simulink model "buildingEnergyManagement"  (R2019b)
settings: Solver=FixedStepAuto  StartTime=0.0  StopTime=24  FixedStep=1/12  RelTol=1e-3  AbsTol=1e-6
values from neighbouring files (symbols this model uses):
  c = 1005.4    [init_vars.m]
  cost = 0.09/3.6e6    (= 2.5e-08)    [init_vars.m]
  eta_ac = 0.85    [init_vars.m]
  initToutdoor = 60    [bonsaiAssess.m]    (also in bonsaiExportConnect.m; bonsaiPredict.m; run_benchmark.m = 30)
  Mdot = 3600    [init_vars.m]
  THeater = 50    [init_vars.m]
  TinIC = 20    [init_vars.m]
undefined symbols (not defined in the file or in its folder): dTac, n_rooms, nWindows_room1, nWindows_room2, nWindows_room3, sigbuilder_block
libraries: simulink_extras x7, bonsai_library x1
Description:
  | Thermal Model of a House
  | 
  | This demo illustrates how you can use Simulink(R) to create the thermal model of
  | a house. This system models the outdoor environment, the thermal
  | characteristics of the house, and the house heating system.
  | 
  | The sldemo_househeat_data.m file initializes data in the model workspace.
  | To make changes, you can edit the model workspace directly or edit the MATLAB(R) file
  | and re-load the model workspace.
  | 
  | To view the model workspace, select View > Model Explorer
  | from the Simulink editor.
  | 
  | Note: Time is given in units of hours
settings Model: ExtModeTrigMode=oneshot  ExtModeArmWhenConnect=off  ExtModeAutoUpdateStatusClock=off  OrderedModelArguments=off  Creator=The MathWorks, Inc.  LastModifiedBy=jomcdowe
settings SolverCC: AutoScaleAbsTol=off
settings DataIOCC: ExternalInput=[]  InitialState=[]  SaveOutput=off  ReturnWorkspaceOutputs=off  SignalLoggingName=sldemo_househeat_output  ReturnWorkspaceOutputsName=simout
settings OptimizationCC: BlockReduction=off  BooleanDataType=off  ExpressionDepthLimit=2147483647  InitFltsAndDblsToZero=on  LifeSpan=inf  BufferReusableBoundary=off
settings DebuggingCC: SaveWithParameterizedLinksMsg=none  UnderspecifiedInitializationDetection=Classic  MergeDetectMultiDrivingBlocksExec=none  SignalResolutionControl=TryResolveAllWithWarning  MultiTaskDSMMsg=warning  MultiTaskCondExecSysMsg=none  IntegerOverflowMsg=none  FcnCallInpInsideContextMsg=warning  BusObjectLabelMismatch=none  StateNameClashWarn=warning  SFUnexpectedBacktrackingDiag=warning  SFNoUnconditionalDefaultTransitionDiag=warning  SFExecutionAtInitializationDiag=none  IntegerSaturationMsg=none  ArithmeticOperatorsInVariantConditions=warning
settings HardwareCC: ProdBitPerPointer=32  ProdBitPerSizeT=32  ProdBitPerPtrDiffT=32  ProdLargestAtomicFloat=None  ProdIntDivRoundTo=Undefined  ProdEndianess=Unspecified  ProdWordSize=32  ProdHWDeviceType=32-bit Generic  TargetUnknown=on
settings ModelReferenceCC: PropagateSignalLabelsOutOfModel=off
settings SFSimCC: SimUseLocalCustomCode=off  CustomCodeUndefinedFunction=UseInterfaceOnly
settings RTWCC: Description=Generic Real-Time Target  RTWUseLocalCustomCode=off
settings CodeAppCC: StateflowObjectComments=on
settings GRTTargetCC: TargetFcnLib=ansi_tfl_tmw.mat  TargetLangStandard=C89/C90 (ANSI)  CombineOutputUpdateFcns=off  GRTInterface=on
settings ConfigComp: CovMetricSettings=dw  CovSaveCumulativeToWorkspaceVar=on  CovSaveSingleToWorkspaceVar=on  CovExternalEMLEnable=off

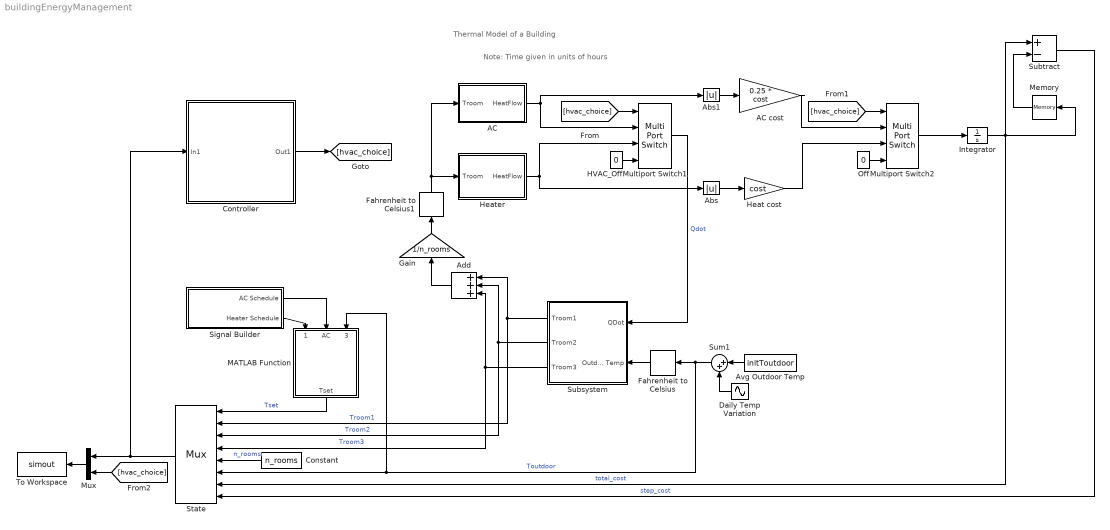
== system buildingEnergyManagement ==
  note: Thermal Model of a Building
  note: Note: Time given in units of hours
  AC : Subsystem
  AC cost : Gain  Gain=0.25 * cost  SaturateOnIntegerOverflow=on  OutDataTypeStr=Inherit: Same as input  ParamDataTypeStr=Inherit: Same as input
  Abs : Abs
  Abs1 : Abs
  Add : Sum  Inputs=+++
  Avg Outdoor Temp : Constant  Value=initToutdoor
  Constant : Constant  Value=n_rooms
  Controller : Subsystem  VariantControlMode=Label  Variant=on  LabelModeActiveChoice=Bonsai  mask{VChoice=Bonsai}
      mask prompts: VChoice "Source"
      mask init:
      | simulationStatus =  get_param(bdroot,'SimulationStatus');
      | 
      | % The active variant can only be modified at edit-time or very early during
      | % the simulink compile stage. 
      | 
      |     choice = get_param(gcb,'VChoice');
      |     vssBlk = gcb;
      |     oldVariant = get_param(gcb,'OverrideUsingVariant');
      | 
      |     if strcmp(choice,'Thermostat')
      |         set_param(vssBlk, 'OverrideUsingVariant', 'Thermostat');
      |     else
      |         set_param(vssBlk, 'OverrideUsingVariant', 'Bonsai');
      |     end
      mask TypeOptions VChoice: Thermostat | Bonsai
      mask Display:
      | choice = get_param(gcb,'VChoice');
      | 
      | if strcmp(choice,'Thermostat')
      |     image('img/Thermostat.jpg');
      | else
      |     image('img/Bonsai.jpg');
      | end
  Daily Temp Variation : Sin  Amplitude=15  Frequency=2*pi/24  SampleTime=0
  Fahrenheit to Celsius : simulink_extras/Transformations/Fahrenheit to Celsius
      settings: SourceProductName=Simulink Extras
  Fahrenheit to Celsius1 : simulink_extras/Transformations/Fahrenheit to Celsius
      settings: SourceProductBaseCode=SL
  Gain : Gain  Gain=1/n_rooms
  HVAC_Off : Constant  Value=0
  "Heat cost " : Gain  Gain=cost  SaturateOnIntegerOverflow=on  OutDataTypeStr=Inherit: Same as input  ParamDataTypeStr=Inherit: Same as input
  Heater : Subsystem
  Integrator : Integrator
  MATLAB Function : MATLAB Function  TreatAsAtomicUnit=on
  Memory : Memory
  Multiport Switch1 : MultiPortSwitch  DiagnosticForDefault=None
  Multiport Switch2 : MultiPortSwitch  DiagnosticForDefault=None
  Mux : Mux  Inputs=2
  Off : Constant  Value=0
  Signal Builder : Subsystem  Tag=STV Subsys  LoadFcn=sigbuilder_block('load');  StartFcn=sigbuilder_block('start');  StopFcn=sigbuilder_block('stop');  ClipboardFcn=sigbuilder_block('clipboard');  mask(Sigbuilder block){tuvar=[0:10]}
      mask help: Simulink:masks:SigbuilderBlock_MD
      mask init:
      | if ~strcmp(get_param(bdroot(gcbh),'SimulationStatus'),'stopped') tuvar = sigbuilder_block('maskInit'); end
      settings: CopyFcn=sigbuilder_block('copy');  DeleteFcn=sigbuilder_block('delete');  ModelCloseFcn=sigbuilder_block('modelClose');  PreSaveFcn=sigbuilder_block('preSave');  PauseFcn=sigbuilder_block('pause');  ContinueFcn=sigbuilder_block('continue');  NameChangeFcn=sigbuilder_block('namechange');  OpenFcn=sigbuilder_block('open',[437.6 199.2 550.4 400 ]);  CloseFcn=sigbuilder_block('close');
      mask Display: plot(0, 0, 100, 100,[2, 2, 32, 32, 2], [68, 8, 8, 68, 68],[32, 2], [38, 38], [32, 19, 2],[53, 60, 44], [32, 17, 17, 2],[16, 16, 31, 31]);txt = getActiveGroup(gcbh);text(2, 100, txt,'verticalAlignment', 'top');
  State : Mux  Inputs=8
      settings: DisplayOption=signals
  Subsystem : Subsystem
  Subtract : Sum  Inputs=+-
  Sum1 : Sum  Inputs=|++  SaturateOnIntegerOverflow=on  InputSameDT=on  OutDataTypeStr=Inherit: Same as first input
  To Workspace : ToWorkspace  VariableName=simout  SampleTime=-1
  wires:
  Sum1/1 -> State/6, MATLAB Function/3(Toutdoor), Fahrenheit to Celsius/1  "Toutdoor"
  Avg Outdoor Temp/1 -> Sum1/1
  Daily Temp Variation/1 -> Sum1/2
  HVAC_Off/1 -> Multiport Switch1/4
  [hvac_choice] -> Multiport Switch1/1
  [hvac_choice] -> Multiport Switch2/1
  Off/1 -> Multiport Switch2/4
  AC/1(HeatFlow) -> Abs1/1, Multiport Switch1/2
  Heater/1(HeatFlow) -> Abs/1, Multiport Switch1/3
  Abs1/1 -> AC cost/1
  Abs/1 -> "Heat cost "/1
  AC cost/1 -> Multiport Switch2/2
  "Heat cost "/1 -> Multiport Switch2/3
  Controller/1(Out1) -> [hvac_choice]
  [hvac_choice] -> Mux/2
  Mux/1 -> To Workspace/1
  Signal Builder/2(Heater Schedule) -> MATLAB Function/1(Heater)
  Signal Builder/1(AC Schedule) -> MATLAB Function/2(AC)
  Multiport Switch1/1 -> Subsystem/1(QDot)  "Qdot"
  Fahrenheit to Celsius/1 -> Subsystem/2(Outdoor Temp)
  State/1 -> Mux/1, Controller/1(In1)
  MATLAB Function/1(Tset) -> State/1  "Tset"
  Integrator/1 -> Memory/1, State/7, Subtract/1  "total_cost"
  Subsystem/1(Troom1) -> Add/1, State/2  "Troom1"
  Subsystem/2(Troom2) -> Add/2, State/3  "Troom2"
  Subsystem/3(Troom3) -> Add/3, State/4  "Troom3"
  Add/1 -> Gain/1
  Fahrenheit to Celsius1/1 -> AC/1(Troom), Heater/1(Troom)
  Gain/1 -> Fahrenheit to Celsius1/1
  Constant/1 -> State/5  "n_rooms"
  Multiport Switch2/1 -> Integrator/1
  Memory/1 -> Subtract/2
  Subtract/1 -> State/8  "step_cost"

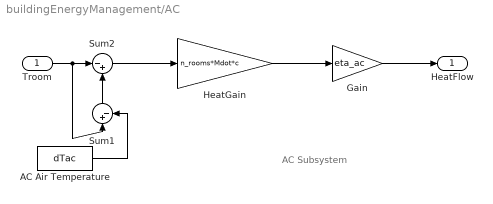
== system buildingEnergyManagement/AC ==
  note: AC Subsystem
  Troom : Inport
  AC Air Temperature : Constant  Value=dTac
  Gain : Gain  Gain=eta_ac
  HeatGain : Gain  Gain=n_rooms*Mdot*c
  Sum1 : Sum  Inputs=|+-
  Sum2 : Sum  Inputs=|-+
  HeatFlow : Outport  VectorParamsAs1DForOutWhenUnconnected=off
  wires:
  Sum2/1 -> HeatGain/1
  Gain/1 -> HeatFlow/1
  HeatGain/1 -> Gain/1
  AC Air Temperature/1 -> Sum1/2
  Troom/1 -> Sum2/1, Sum1/1
  Sum1/1 -> Sum2/2

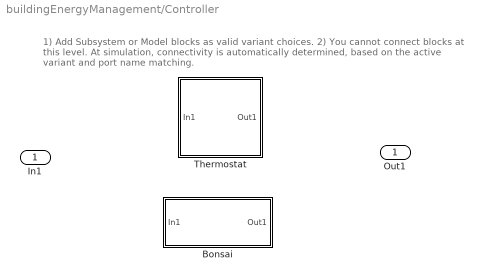
== system buildingEnergyManagement/Controller ==
  note: 1) Add Subsystem or Model blocks as valid variant choices.
      | 2) You cannot connect blocks at this level. At simulation, connectivity is automatically
      | determined, based on the active variant and port name matching.
  In1 : Inport
  Bonsai : Subsystem  VariantControl=Bonsai
  Thermostat : Subsystem  VariantControl=Thermostat
      mask Display: image(fullfile(matlabroot,'toolbox','simulink','simdemos','simgeneral','images','HouseHeatThermostatPix.svg'))
  Out1 : Outport

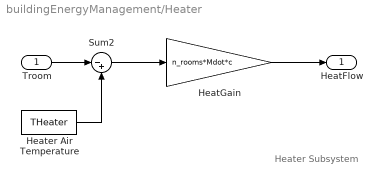
== system buildingEnergyManagement/Heater ==
  note: Heater Subsystem
  Troom : Inport
  HeatGain : Gain  Gain=n_rooms*Mdot*c
  Heater Air Temperature : Constant  Value=THeater
  Sum2 : Sum  Inputs=|-+
  HeatFlow : Outport  VectorParamsAs1DForOutWhenUnconnected=off
  wires:
  Heater Air Temperature/1 -> Sum2/2
  Troom/1 -> Sum2/1
  Sum2/1 -> HeatGain/1
  HeatGain/1 -> HeatFlow/1

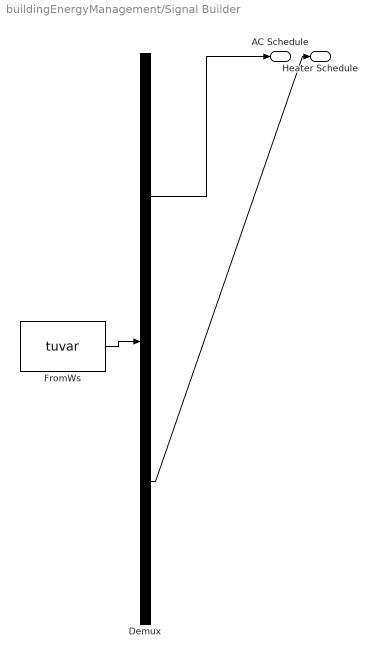
== system buildingEnergyManagement/Signal Builder ==
  Demux : Demux  Tag=STV Demux  Outputs=2
  FromWs : FromWorkspace  Tag=STV FromWs  VariableName=tuvar  SampleTime=0
      SigBuilderData=|
      | common.afterFinalStr = 'Extrapolate'
      | common.sampleTime = 0
      | dataSet.timeRange = [0 24]
      | dataSet.name = 'Tset_choice'
      | sbobj.Groups.Name = 'Tset_choice'
      | sbobj.Groups.Signals(1).Name = 'AC Schedule'
      | sbobj.Groups.Signals(1).XData = [0 12 12 24]
      | sbobj.Groups.Signals(1).YData = [78 78 86 86]
      | sbobj.Groups.Signals(2).Name = 'Heater Schedule'
      | sbobj.Groups.Signals(2).XData = [0 12 12 24]
      | sbobj.Groups.Signals(2).YData = [68 68 60 60]
      | sbobj.Groups.TimeRange = [0 24]
  AC Schedule : Outport  Tag=STV Outport
  Heater Schedule : Outport  Tag=STV Outport  Port=2
  wires:
  Demux/1 -> AC Schedule/1
  FromWs/1 -> Demux/1
  Demux/2 -> Heater Schedule/1

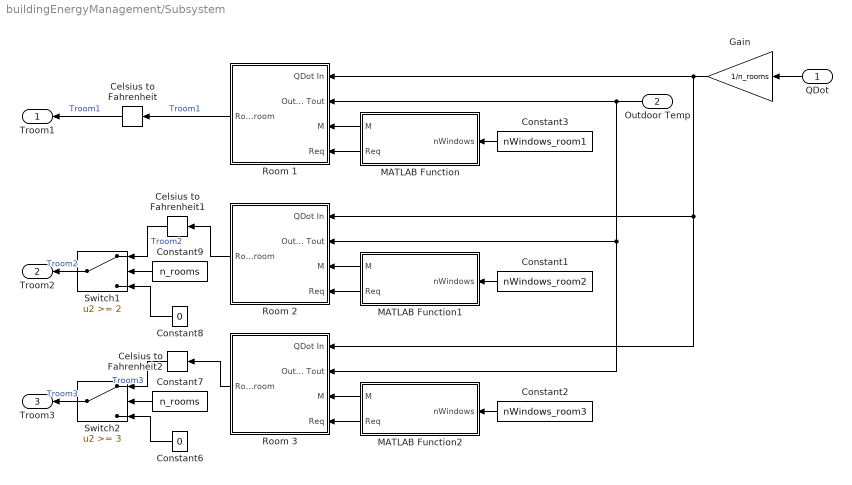
== system buildingEnergyManagement/Subsystem ==
  QDot : Inport
  Outdoor Temp : Inport  Port=2
  Celsius to Fahrenheit : simulink_extras/Transformations/Celsius to Fahrenheit
      settings: SourceProductName=Simulink Extras
  Celsius to Fahrenheit1 : simulink_extras/Transformations/Celsius to Fahrenheit
      settings: SourceProductName=Simulink Extras
  Celsius to Fahrenheit2 : simulink_extras/Transformations/Celsius to Fahrenheit
      settings: SourceProductName=Simulink Extras
  Constant1 : Constant  Value=nWindows_room2  VectorParams1D=off
  Constant2 : Constant  Value=nWindows_room3  VectorParams1D=off
  Constant3 : Constant  Value=nWindows_room1  VectorParams1D=off
  Constant6 : Constant  Value=0
  Constant7 : Constant  Value=n_rooms
  Constant8 : Constant  Value=0
  Constant9 : Constant  Value=n_rooms
  Gain : Gain  Gain=1/n_rooms
  MATLAB Function : MATLAB Function  TreatAsAtomicUnit=on
  MATLAB Function1 : MATLAB Function  TreatAsAtomicUnit=on
  MATLAB Function2 : MATLAB Function  TreatAsAtomicUnit=on
  Room 1 : Subsystem
      mask Display: image(fullfile(matlabroot,'toolbox','simulink','simdemos','simgeneral','images','HouseHeatHousePix.svg'))
  Room 2 : Subsystem
      mask Display: image(fullfile(matlabroot,'toolbox','simulink','simdemos','simgeneral','images','HouseHeatHousePix.svg'))
  Room 3 : Subsystem
      mask Display: image(fullfile(matlabroot,'toolbox','simulink','simdemos','simgeneral','images','HouseHeatHousePix.svg'))
  Switch1 : Switch  Threshold=2
  Switch2 : Switch  Threshold=3
  Troom1 : Outport
  Troom2 : Outport  Port=2
  Troom3 : Outport  Port=3
  wires:
  Gain/1 -> Room 1/1(QDot In), Room 2/1(QDot In), Room 3/1(QDot In)
  Outdoor Temp/1 -> Room 1/2(Outdoor Temp Tout), Room 2/2(Outdoor Temp Tout), Room 3/2(Outdoor Temp Tout)
  QDot/1 -> Gain/1
  Constant9/1 -> Switch1/2
  Room 2/1(Room Temp Troom) -> Celsius to Fahrenheit1/1
  Constant7/1 -> Switch2/2
  Room 3/1(Room Temp Troom) -> Celsius to Fahrenheit2/1
  Switch2/1 -> Troom3/1  "Troom3"
  Switch1/1 -> Troom2/1  "Troom2"
  Room 1/1(Room Temp Troom) -> Celsius to Fahrenheit/1  "Troom1"
  Celsius to Fahrenheit/1 -> Troom1/1  "Troom1"
  Constant8/1 -> Switch1/3
  Celsius to Fahrenheit1/1 -> Switch1/1  "Troom2"
  Celsius to Fahrenheit2/1 -> Switch2/1  "Troom3"
  Constant6/1 -> Switch2/3
  MATLAB Function/1(M) -> Room 1/3(M)
  MATLAB Function/2(Req) -> Room 1/4(Req)
  Constant3/1 -> MATLAB Function/1(nWindows)
  MATLAB Function1/1(M) -> Room 2/3(M)
  MATLAB Function1/2(Req) -> Room 2/4(Req)
  Constant1/1 -> MATLAB Function1/1(nWindows)
  MATLAB Function2/1(M) -> Room 3/3(M)
  MATLAB Function2/2(Req) -> Room 3/4(Req)
  Constant2/1 -> MATLAB Function2/1(nWindows)

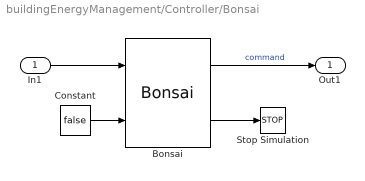
== system buildingEnergyManagement/Controller/Bonsai ==
  In1 : Inport
  Bonsai : bonsai_library/Bonsai  sampleTime=[-1, 0]
      settings: SourceProductName=Bonsai Toolbox
  Constant : Constant  Value=false
  Stop Simulation : Stop
  Out1 : Outport
  wires:
  Bonsai/1 -> Out1/1  "command"
  In1/1 -> Bonsai/1
  Constant/1 -> Bonsai/2
  Bonsai/2 -> Stop Simulation/1

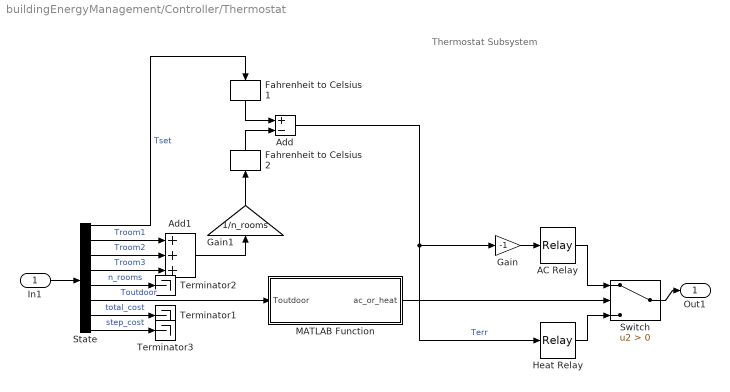
== system buildingEnergyManagement/Controller/Thermostat ==
  note: Thermostat Subsystem
  In1 : Inport
  AC Relay : Relay  OnSwitchValue=5*(5/9)  OffSwitchValue=-5*(5/9)  OffOutputValue=3
  Add : Sum  Inputs=+-
  Add1 : Sum  Inputs=+++
  Fahrenheit to Celsius 1 : simulink_extras/Transformations/Fahrenheit to Celsius
      settings: SourceProductName=Simulink Extras
  Fahrenheit to Celsius 2 : simulink_extras/Transformations/Fahrenheit to Celsius
      settings: SourceProductName=Simulink Extras
  Gain : Gain  Gain=-1
  Gain1 : Gain  Gain=1/n_rooms
  Heat Relay : Relay  OnSwitchValue=5*(5/9)  OffSwitchValue=-5*(5/9)  OnOutputValue=2  OffOutputValue=3
  MATLAB Function : MATLAB Function  TreatAsAtomicUnit=on
  State : Demux  Outputs=8
  Switch : Switch  Criteria=u2 > Threshold
  Terminator1 : Terminator
  Terminator2 : Terminator
  Terminator3 : Terminator
  Out1 : Outport
  wires:
  Add/1 -> Heat Relay/1, Gain/1  "Terr"
  MATLAB Function/1(ac_or_heat) -> Switch/2
  Heat Relay/1 -> Switch/3
  AC Relay/1 -> Switch/1
  Switch/1 -> Out1/1
  Gain/1 -> AC Relay/1
  Fahrenheit to Celsius 1/1 -> Add/1
  Fahrenheit to Celsius 2/1 -> Add/2
  In1/1 -> State/1
  State/1 -> Fahrenheit to Celsius 1/1  "Tset"
  State/3 -> Add1/2  "Troom2"
  State/4 -> Add1/3  "Troom3"
  State/2 -> Add1/1  "Troom1"
  Add1/1 -> Gain1/1
  Gain1/1 -> Fahrenheit to Celsius 2/1
  State/7 -> Terminator1/1  "total_cost"
  State/6 -> MATLAB Function/1(Toutdoor)  "Toutdoor"
  State/5 -> Terminator2/1  "n_rooms"
  State/8 -> Terminator3/1  "step_cost"

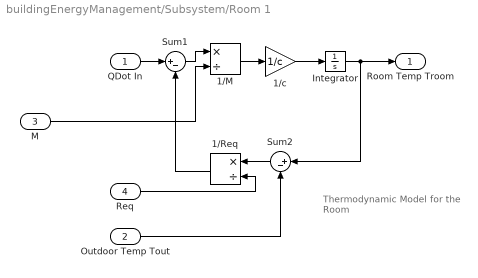
== system buildingEnergyManagement/Subsystem/Room 1 ==
  note: Thermodynamic Model
      | for the Room
  QDot In : Inport
  Outdoor Temp Tout : Inport  Port=2
  M : Inport  Port=3
  Req : Inport  Port=4
  1/M : Product  Inputs=*/
  1/Req : Product  Inputs=*/
  1/c : Gain  Gain=1/c  SaturateOnIntegerOverflow=on  OutDataTypeStr=Inherit: Same as input  ParamDataTypeStr=Inherit: Same as input
  Integrator : Integrator  InitialCondition=TinIC
  Sum1 : Sum  Inputs=|+-  SaturateOnIntegerOverflow=on  InputSameDT=on  OutDataTypeStr=Inherit: Same as first input
  Sum2 : Sum  Inputs=|+-  SaturateOnIntegerOverflow=on  InputSameDT=on  OutDataTypeStr=Inherit: Same as first input
  Room Temp Troom : Outport  InitialOutput=0  VectorParamsAs1DForOutWhenUnconnected=off
  wires:
  M/1 -> 1/M/2
  1/M/1 -> 1/c/1
  Sum1/1 -> 1/M/1
  Req/1 -> 1/Req/2
  Integrator/1 -> Room Temp Troom/1, Sum2/1
  1/c/1 -> Integrator/1
  1/Req/1 -> Sum1/2
  Sum2/1 -> 1/Req/1
  QDot In/1 -> Sum1/1
  Outdoor Temp Tout/1 -> Sum2/2

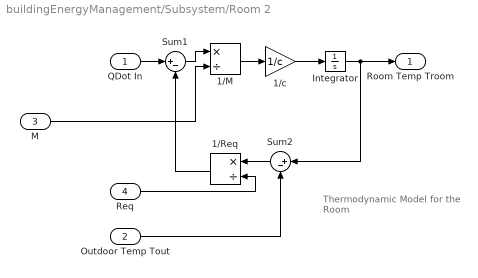
== system buildingEnergyManagement/Subsystem/Room 2 ==
  note: Thermodynamic Model
      | for the Room
  QDot In : Inport
  Outdoor Temp Tout : Inport  Port=2
  M : Inport  Port=3
  Req : Inport  Port=4
  1/M : Product  Inputs=*/
  1/Req : Product  Inputs=*/
  1/c : Gain  Gain=1/c  SaturateOnIntegerOverflow=on  OutDataTypeStr=Inherit: Same as input  ParamDataTypeStr=Inherit: Same as input
  Integrator : Integrator  InitialCondition=TinIC
  Sum1 : Sum  Inputs=|+-  SaturateOnIntegerOverflow=on  InputSameDT=on  OutDataTypeStr=Inherit: Same as first input
  Sum2 : Sum  Inputs=|+-  SaturateOnIntegerOverflow=on  InputSameDT=on  OutDataTypeStr=Inherit: Same as first input
  Room Temp Troom : Outport  InitialOutput=0  VectorParamsAs1DForOutWhenUnconnected=off
  wires:
  M/1 -> 1/M/2
  1/M/1 -> 1/c/1
  Sum1/1 -> 1/M/1
  Req/1 -> 1/Req/2
  Integrator/1 -> Room Temp Troom/1, Sum2/1
  1/c/1 -> Integrator/1
  1/Req/1 -> Sum1/2
  Sum2/1 -> 1/Req/1
  QDot In/1 -> Sum1/1
  Outdoor Temp Tout/1 -> Sum2/2

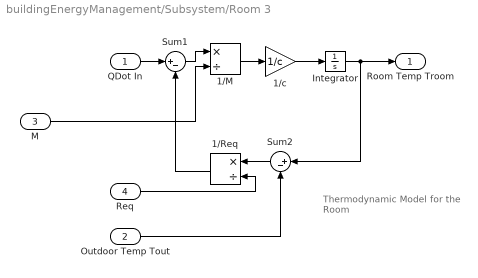
== system buildingEnergyManagement/Subsystem/Room 3 ==
  note: Thermodynamic Model
      | for the Room
  QDot In : Inport
  Outdoor Temp Tout : Inport  Port=2
  M : Inport  Port=3
  Req : Inport  Port=4
  1/M : Product  Inputs=*/
  1/Req : Product  Inputs=*/
  1/c : Gain  Gain=1/c  SaturateOnIntegerOverflow=on  OutDataTypeStr=Inherit: Same as input  ParamDataTypeStr=Inherit: Same as input
  Integrator : Integrator  InitialCondition=TinIC
  Sum1 : Sum  Inputs=|+-  SaturateOnIntegerOverflow=on  InputSameDT=on  OutDataTypeStr=Inherit: Same as first input
  Sum2 : Sum  Inputs=|+-  SaturateOnIntegerOverflow=on  InputSameDT=on  OutDataTypeStr=Inherit: Same as first input
  Room Temp Troom : Outport  InitialOutput=0  VectorParamsAs1DForOutWhenUnconnected=off
  wires:
  M/1 -> 1/M/2
  1/M/1 -> 1/c/1
  Sum1/1 -> 1/M/1
  Req/1 -> 1/Req/2
  Integrator/1 -> Room Temp Troom/1, Sum2/1
  1/c/1 -> Integrator/1
  1/Req/1 -> Sum1/2
  Sum2/1 -> 1/Req/1
  QDot In/1 -> Sum1/1
  Outdoor Temp Tout/1 -> Sum2/2

== matlab function buildingEnergyManagement/MATLAB Function ==
  data: Heater input; AC input; Tset output; Toutdoor input
function Tset = choose_Tset(Heater, AC, Toutdoor)

if Toutdoor > 73
    Tset = AC;
else
    Tset = Heater;
end

== matlab function buildingEnergyManagement/Controller/Thermostat/MATLAB Function ==
  data: Toutdoor input; ac_or_heat output
function ac_or_heat = fcn(Toutdoor)

    if Toutdoor > 73
        ac_or_heat = 1; % AC
    else
        ac_or_heat = -1; % Heat
    end

== matlab function buildingEnergyManagement/Subsystem/MATLAB Function ==
  data: nWindows input; M output; Req output
function [M, Req] = room_params(nWindows)
    % -------------------------------
    % Define the room geometry
    % -------------------------------
    % convert radians to degrees
    r2d = 180/pi;
    % Room length = 30 m
    lenRoom = 30;
    % Room width = 10 m
    widRoom = 10;
    % Room height = 4 m
    htRoom = 4;
    % Roof pitch = 40 deg
    pitRoof = 40/r2d;
    % Number of windows = 6
    numWindows = nWindows;
    % Height of windows = 1 m
    htWindows = 1;
    % Width of windows = 1 m
    widWindows = 1;
    windowArea = numWindows*htWindows*widWindows;
    wallArea = 2*lenRoom*htRoom + 2*widRoom*htRoom + ...
               2*(1/cos(pitRoof/2))*widRoom*lenRoom + ...
               tan(pitRoof)*widRoom - windowArea;
    % -------------------------------
    % Define the type of insulation used
    % -------------------------------
    % Glass wool in the walls, 0.2 m thick
    % k is in units of J/sec/m/C - convert to J/hr/m/C multiplying by 3600
    kWall = 0.038*3600;   % hour is the time unit
    LWall = .2;
    RWall = LWall/(kWall*wallArea);
    % Glass windows, 0.01 m thick
    kWindow = 0.78*3600;  % hour is the time unit
    LWindow = .01;
    RWindow = LWindow/(kWindow*windowArea);
    % -------------------------------
    % Determine the equivalent thermal resistance for the whole building
    % -------------------------------
    Req = RWall*RWindow/(RWall + RWindow);
    % -------------------------------
    % Determine total internal air mass = M
    % -------------------------------
    % Density of air at sea level = 1.2250 kg/m^3
    densAir = 1.2250;
    M = (lenRoom*widRoom*htRoom+tan(pitRoof)*widRoom*lenRoom)*densAir;
end

== matlab function buildingEnergyManagement/Subsystem/MATLAB Function1 ==
  data: nWindows input; M output; Req output
function [M, Req] = room_params(nWindows)
    % -------------------------------
    % Define the room geometry
    % -------------------------------
    % convert radians to degrees
    r2d = 180/pi;
    % Room length = 30 m
    lenRoom = 30;
    % Room width = 10 m
    widRoom = 10;
    % Room height = 4 m
    htRoom = 4;
    % Roof pitch = 40 deg
    pitRoof = 40/r2d;
    % Number of windows = 6
    numWindows = nWindows;
    % Height of windows = 1 m
    htWindows = 1;
    % Width of windows = 1 m
    widWindows = 1;
    windowArea = numWindows*htWindows*widWindows;
    wallArea = 2*lenRoom*htRoom + 2*widRoom*htRoom + ...
               2*(1/cos(pitRoof/2))*widRoom*lenRoom + ...
               tan(pitRoof)*widRoom - windowArea;
    % -------------------------------
    % Define the type of insulation used
    % -------------------------------
    % Glass wool in the walls, 0.2 m thick
    % k is in units of J/sec/m/C - convert to J/hr/m/C multiplying by 3600
    kWall = 0.038*3600;   % hour is the time unit
    LWall = .2;
    RWall = LWall/(kWall*wallArea);
    % Glass windows, 0.01 m thick
    kWindow = 0.78*3600;  % hour is the time unit
    LWindow = .01;
    RWindow = LWindow/(kWindow*windowArea);
    % -------------------------------
    % Determine the equivalent thermal resistance for the whole building
    % -------------------------------
    Req = RWall*RWindow/(RWall + RWindow);
    % -------------------------------
    % Determine total internal air mass = M
    % -------------------------------
    % Density of air at sea level = 1.2250 kg/m^3
    densAir = 1.2250;
    M = (lenRoom*widRoom*htRoom+tan(pitRoof)*widRoom*lenRoom)*densAir;
end

== matlab function buildingEnergyManagement/Subsystem/MATLAB Function2 ==
  data: nWindows input; M output; Req output
function [M, Req] = room_params(nWindows)
    % -------------------------------
    % Define the room geometry
    % -------------------------------
    % convert radians to degrees
    r2d = 180/pi;
    % Room length = 30 m
    lenRoom = 30;
    % Room width = 10 m
    widRoom = 10;
    % Room height = 4 m
    htRoom = 4;
    % Roof pitch = 40 deg
    pitRoof = 40/r2d;
    % Number of windows = 6
    numWindows = nWindows;
    % Height of windows = 1 m
    htWindows = 1;
    % Width of windows = 1 m
    widWindows = 1;
    windowArea = numWindows*htWindows*widWindows;
    wallArea = 2*lenRoom*htRoom + 2*widRoom*htRoom + ...
               2*(1/cos(pitRoof/2))*widRoom*lenRoom + ...
               tan(pitRoof)*widRoom - windowArea;
    % -------------------------------
    % Define the type of insulation used
    % -------------------------------
    % Glass wool in the walls, 0.2 m thick
    % k is in units of J/sec/m/C - convert to J/hr/m/C multiplying by 3600
    kWall = 0.038*3600;   % hour is the time unit
    LWall = .2;
    RWall = LWall/(kWall*wallArea);
    % Glass windows, 0.01 m thick
    kWindow = 0.78*3600;  % hour is the time unit
    LWindow = .01;
    RWindow = LWindow/(kWindow*windowArea);
    % -------------------------------
    % Determine the equivalent thermal resistance for the whole building
    % -------------------------------
    Req = RWall*RWindow/(RWall + RWindow);
    % -------------------------------
    % Determine total internal air mass = M
    % -------------------------------
    % Density of air at sea level = 1.2250 kg/m^3
    densAir = 1.2250;
    M = (lenRoom*widRoom*htRoom+tan(pitRoof)*widRoom*lenRoom)*densAir;
end
